simulink model "simulationTask2_3"  (R2024a)
settings: Solver=VariableStepAuto  StartTime=0.0  StopTime=10  RelTol=1e-3
InitFcn:
  | m1 = 290;
  | b1 = 1000;
  | m2 = 59;
  | k1 = 16182;
  | f = 0;
  | k2 = 19000;
libraries: fl_lib x11, nesl_utility x4

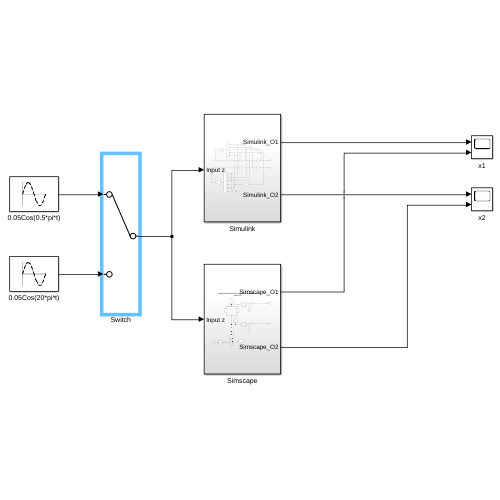
[thumbnail: Simulink's stored preview of the top-level diagram]
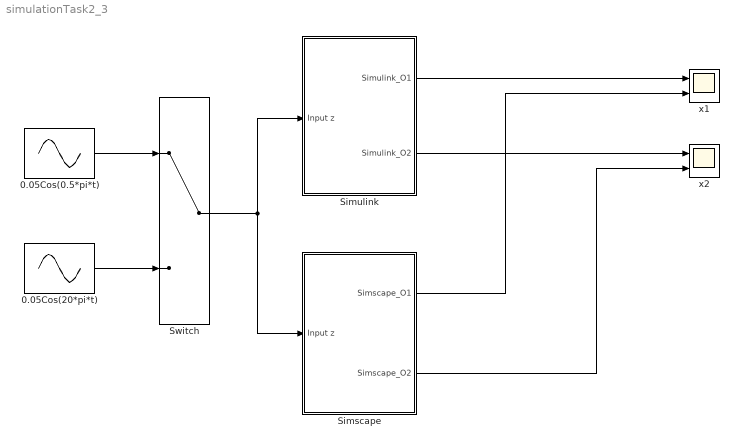
== system simulationTask2_3 ==
  0.05Cos(0.5*pi*t) : Sin  Amplitude=0.05  Frequency=0.5*pi  SampleTime=0
  0.05Cos(20*pi*t) : Sin  Amplitude=0.05  Frequency=20*pi  SampleTime=0
  Simscape : Subsystem
  Simulink : Subsystem
  Switch : ManualSwitch
  x1 : Scope  NumInputPorts=2
  x2 : Scope  NumInputPorts=2
  wires:
  0.05Cos(20*pi*t)/1 -> Switch/2
  Simulink/2(Simulink_O2) -> x2/1
  0.05Cos(0.5*pi*t)/1 -> Switch/1
  Switch/1 -> Simscape/1(Input z), Simulink/1(Input z)
  Simscape/2(Simscape_O2) -> x2/2
  Simulink/1(Simulink_O1) -> x1/1
  Simscape/1(Simscape_O1) -> x1/2

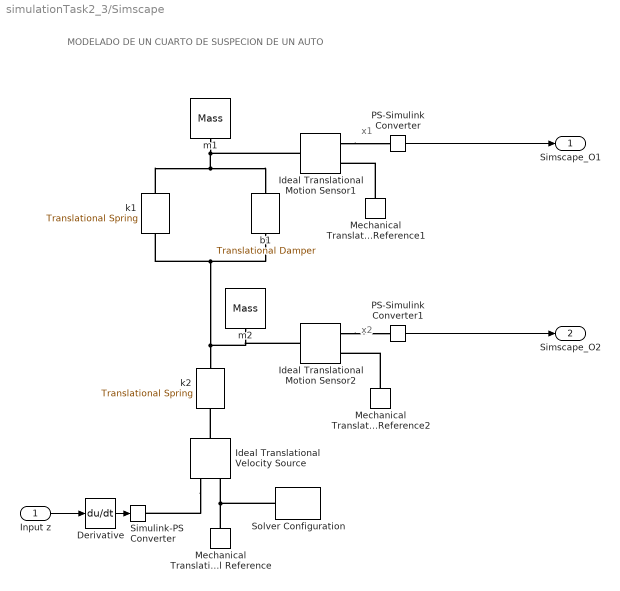
== system simulationTask2_3/Simscape ==
  note: MODELADO DE UN CUARTO DE SUSPECION DE UN AUTO
  note: x2
  note: x1
  Input z : Inport
  Derivative : Derivative
  Ideal Translational Motion Sensor1 : fl_lib/Mechanical/Mechanical Sensors/Ideal Translational Motion Sensor  reference=foundation.enum.MeasurementReference.difference  acceleration_port=false  velocity_port=false  position_port=true  offset=0 m
      settings: InternalSimscapePortConfiguration="{\"Bottom\":[],\"Left\":[{\"id\":\"R\",\"label\":\"R\",\"type\":\"foundation.mechanical.translational.translational\"}],\"Right\":[{\"id\":\"C\",\"label\":\"C\",\"type\":\"foundation.mechanical.translational.translational\"},{\"id\":\"P\",\"label\":\"P\",\"type\":\"output\"}],\"Top\":[]}"
  Ideal Translational Motion Sensor2 : fl_lib/Mechanical/Mechanical Sensors/Ideal Translational Motion Sensor  reference=foundation.enum.MeasurementReference.difference  acceleration_port=false  velocity_port=false  position_port=true  offset=0 m
      settings: InternalSimscapePortConfiguration="{\"Bottom\":[],\"Left\":[{\"id\":\"R\",\"label\":\"R\",\"type\":\"foundation.mechanical.translational.translational\"}],\"Right\":[{\"id\":\"C\",\"label\":\"C\",\"type\":\"foundation.mechanical.translational.translational\"},{\"id\":\"P\",\"label\":\"P\",\"type\":\"output\"}],\"Top\":[]}"
  Ideal Translational Velocity Source : fl_lib/Mechanical/Mechanical Sources/Ideal Translational Velocity Source
  Mechanical Translational Reference : fl_lib/Mechanical/Translational Elements/Mechanical Translational Reference
  Mechanical Translational Reference1 : fl_lib/Mechanical/Translational Elements/Mechanical Translational Reference
  Mechanical Translational Reference2 : fl_lib/Mechanical/Translational Elements/Mechanical Translational Reference
  PS-Simulink Converter : nesl_utility/PS-Simulink Converter  PhysicalDomain=network_engine_domain  SubClassName=ps_output  LeftPortType=input  RightPortType=output  PseudoPeriodic=off  Frequencies=[]  VectorFormat=inherit  Unit=inherit  AffineConversion=off
  PS-Simulink Converter1 : nesl_utility/PS-Simulink Converter  PhysicalDomain=network_engine_domain  SubClassName=ps_output  LeftPortType=input  RightPortType=output  PseudoPeriodic=off  Frequencies=[]  VectorFormat=inherit  Unit=inherit  AffineConversion=off
  Simulink-PS Converter : nesl_utility/Simulink-PS Converter  PhysicalDomain=network_engine_domain  SubClassName=ps_input  LeftPortType=input  RightPortType=output  PseudoPeriodic=off  Frequencies=[]  NoiseDistribution=none  NoiseParameters=[]  Unit=1  AffineConversion=off  FilteringAndDerivatives=provide  SimscapeFilterOrder=1  InputFilterTimeConstant=0.001  UdotUserProvided=0
  Solver Configuration : nesl_utility/Solver Configuration  PhysicalDomain=network_engine_domain  SubClassName=solver  LeftPortType=input  RightPortType=generic  Tones=[]  Harmonics=[]  SimulateNoise=off  Profile=off  UseLocalSampling=off  EnableSwitchedLinearOptims=on  FrequencyDomain=off  UseCCode=off  RelTol=0.001  AbsTol=0.001  MinStep=1e-09  ToWorkspace=off  RevertToSquareIcSolve=off  NumHomotopyIterations=100  PhasorMode=off  PhasorModeNumHarmonics=1  ConsistencySolver=NEWTON_XTOL_AFTER_FTOL  IndexReductionMethod=DerivativeReplacement  DoDC=off  ResidualTolerance=1e-09  ConsistencyTolSource=GLOBAL  ConsistencyAbsTol=0.001  ConsistencyRelTol=0.001  ConsistencyTolFactor=0.001  UseLocalSolver=on  LocalSolverChoice=NE_BACKWARD_EULER_ADVANCER  ResolveIndetEquations=on  FunctionEvalNumThread=1  LocalSolverSampleTime=0.0001  DoFixedCost=on  MaxNonlinIter=3  MaxModeIter=2  ComputeImpulses=off  ImpulseIterations=2  LinearAlgebra=auto  LinearAlgebraNumThread=0  EquationFormulation=NE_TIME_EF  DelaysMemoryBudget=1024  AutomaticFiltering=on  FilteringTimeConstant=0.001  PartitionStorageMethod=AS_NEEDED  PartitionMemoryBudget=1024  PartitionMethod=ROBUST  MultibodyUseLocalSolver=off  MultibodyLocalSolverChoice=ODE1  MultibodyLocalSolverSampleTime=0.001
  b1 : fl_lib/Mechanical/Translational Elements/Translational Damper  D=b1 N*s/m  v_specify=off  v_priority=None  v=0 m/s  v_nominal_specify=off  v_nominal_value=1  v_nominal_unit=m/s  f_specify=off  f_priority=None  f=0 N  f_nominal_specify=off  f_nominal_value=1  f_nominal_unit=N
  k1 : fl_lib/Mechanical/Translational Elements/Translational Spring  spr_rate=k1 N/m  v_specify=off  v_priority=None  v=0 m/s  v_nominal_specify=off  v_nominal_value=1  v_nominal_unit=m/s  f_specify=off  f_priority=None  f=0 N  f_nominal_specify=off  f_nominal_value=1  f_nominal_unit=N  x_specify=off  x_priority=High  x=0 m  x_nominal_specify=off  x_nominal_value=1  x_nominal_unit=m
  k2 : fl_lib/Mechanical/Translational Elements/Translational Spring  spr_rate=k2 N/m  v_specify=off  v_priority=None  v=0 m/s  v_nominal_specify=off  v_nominal_value=1  v_nominal_unit=m/s  f_specify=off  f_priority=None  f=0 N  f_nominal_specify=off  f_nominal_value=1  f_nominal_unit=N  x_specify=off  x_priority=High  x=0 m  x_nominal_specify=off  x_nominal_value=1  x_nominal_unit=m
  m1 : fl_lib/Mechanical/Translational Elements/Mass  mass=m1 kg  num_ports=foundation.enum.numPorts2.one  v_specify=off  v_priority=High  v=0 m/s  v_nominal_specify=off  v_nominal_value=1  v_nominal_unit=m/s  f_specify=off  f_priority=None  f=0 N  f_nominal_specify=off  f_nominal_value=1  f_nominal_unit=N
  m2 : fl_lib/Mechanical/Translational Elements/Mass  mass=m2 kg  num_ports=foundation.enum.numPorts2.one  v_specify=off  v_priority=High  v=0 m/s  v_nominal_specify=off  v_nominal_value=1  v_nominal_unit=m/s  f_specify=off  f_priority=None  f=0 N  f_nominal_specify=off  f_nominal_value=1  f_nominal_unit=N
  Simscape_O1 : Outport
  Simscape_O2 : Outport  Port=2
  wires:
  PS-Simulink Converter/1 -> Simscape_O1/1
  Input z/1 -> Derivative/1
  Derivative/1 -> Simulink-PS Converter/1
  PS-Simulink Converter1/1 -> Simscape_O2/1
  connections:
  Mechanical Translational Reference1/LConn1 -- Ideal Translational Motion Sensor1/RConn1
  Ideal Translational Velocity Source/LConn1 -- k2/RConn1
  Ideal Translational Motion Sensor1/RConn2 -- PS-Simulink Converter/LConn1
  b1/RConn1 -- k1/RConn1 -- Ideal Translational Motion Sensor2/LConn1 -- m2/LConn1 -- k2/LConn1
  k1/LConn1 -- Ideal Translational Motion Sensor1/LConn1 -- m1/LConn1 -- b1/LConn1
  Mechanical Translational Reference/LConn1 -- Solver Configuration/RConn1 -- Ideal Translational Velocity Source/RConn2
  Ideal Translational Velocity Source/RConn1 -- Simulink-PS Converter/RConn1
  Mechanical Translational Reference2/LConn1 -- Ideal Translational Motion Sensor2/RConn1
  Ideal Translational Motion Sensor2/RConn2 -- PS-Simulink Converter1/LConn1

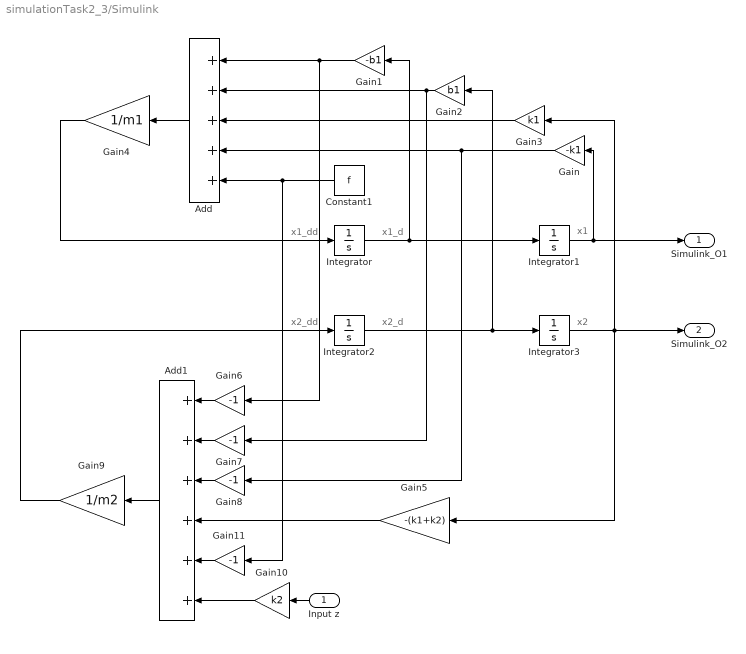
== system simulationTask2_3/Simulink ==
  note: x1
  note: x1_dd
  note: x1_d
  note: x2
  note: x2_d
  note: x2_dd
  Input z : Inport
  Add : Sum  Inputs=+++++
  Add1 : Sum  Inputs=++++++
  Constant1 : Constant  Value=f
  Gain : Gain  Gain=-k1
  Gain1 : Gain  Gain=-b1
  Gain10 : Gain  Gain=k2
  Gain{6..8,11} (4 alike) : Gain  Gain=-1
  Gain2 : Gain  Gain=b1
  Gain3 : Gain  Gain=k1
  Gain4 : Gain  Gain=1/m1
  Gain5 : Gain  Gain=-(k1+k2)
  Gain9 : Gain  Gain=1/m2
  Integrator{,1..3} (4 alike) : Integrator
  Simulink_O1 : Outport
  Simulink_O2 : Outport  Port=2
  wires:
  Gain9/1 -> Integrator2/1
  Gain5/1 -> Add1/4
  Add1/1 -> Gain9/1
  Gain8/1 -> Add1/3
  Gain7/1 -> Add1/2
  Gain3/1 -> Add/3
  Gain10/1 -> Add1/6
  Gain2/1 -> Gain7/1, Add/2
  Constant1/1 -> Gain11/1, Add/5
  Gain4/1 -> Integrator/1
  Integrator1/1 -> Simulink_O1/1, Gain/1
  Input z/1 -> Gain10/1
  Gain11/1 -> Add1/5
  Integrator2/1 -> Integrator3/1, Gain2/1
  Gain1/1 -> Gain6/1, Add/1
  Integrator/1 -> Integrator1/1, Gain1/1
  Integrator3/1 -> Simulink_O2/1, Gain3/1, Gain5/1
  Gain/1 -> Gain8/1, Add/4
  Add/1 -> Gain4/1
  Gain6/1 -> Add1/1
